simulink model "tp1_sim"  (R2018a)
settings: Solver=VariableStepAuto  StartTime=0.0  StopTime=50.0  RelTol=1e-3
values from neighbouring files (symbols this model uses):
  lambda_f = 3    [tp1.m]
  lambda_p = 5    [tp1.m]
settings Model: Creator=e1802460  LastModifiedBy=e1802460

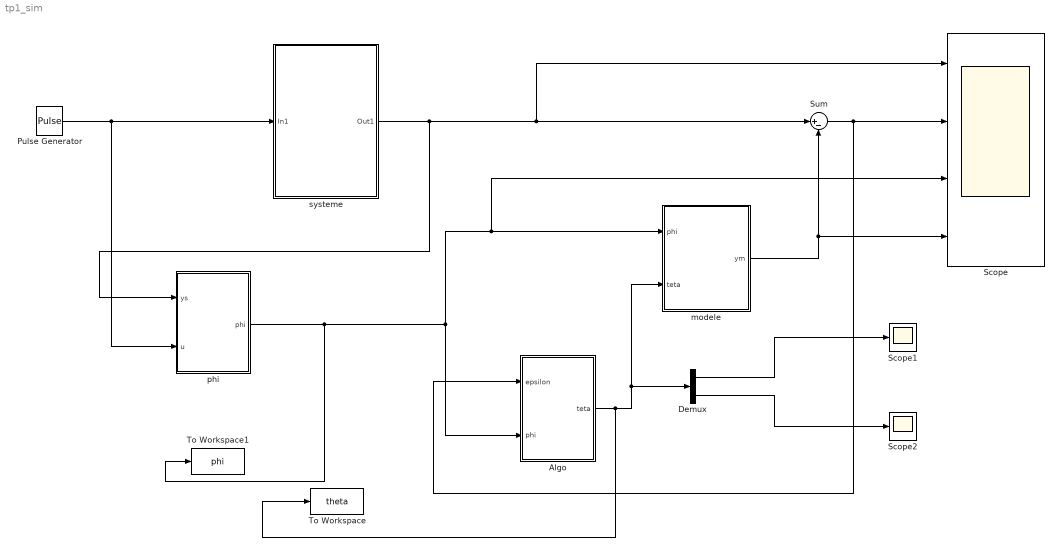
== system tp1_sim ==
  " modele " : Subsystem
  "Algo " : Subsystem
  Demux : Demux  Outputs=2
  Pulse Generator : DiscretePulseGenerator  PulseType=Time based  Period=10  PulseWidth=50
  Scope : Scope  NumInputPorts=4
  Scope1 : Scope
  Scope2 : Scope
  Sum : Sum  Inputs=|+-
  To Workspace : ToWorkspace  VariableName=theta  SaveFormat=Structure With Time  SampleTime=-1
  To Workspace1 : ToWorkspace  VariableName=phi  SaveFormat=Structure With Time  SampleTime=-1
  phi : Subsystem
  "systeme " : Subsystem
  wires:
  "systeme "/1(Out1) -> phi/1(ys), Scope/1, Sum/1
  Pulse Generator/1 -> phi/2(u), "systeme "/1(In1)
  " modele "/1(ym) -> Scope/4, Sum/2
  Sum/1 -> "Algo "/1(epsilon), Scope/2
  phi/1(phi) -> To Workspace1/1, "Algo "/2("phi "), Scope/3, " modele "/1(phi)
  "Algo "/1(teta) -> To Workspace/1, Demux/1, " modele "/2(teta)
  Demux/1 -> Scope1/1
  Demux/2 -> Scope2/1

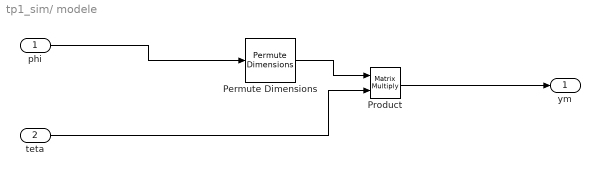
== system tp1_sim/ modele  ==
  phi : Inport
  teta : Inport  Port=2
  Permute Dimensions : PermuteDimensions
  Product : Product  Multiplication=Matrix(*)
  ym : Outport
  wires:
  Permute Dimensions/1 -> Product/1
  phi/1 -> Permute Dimensions/1
  Product/1 -> ym/1
  teta/1 -> Product/2

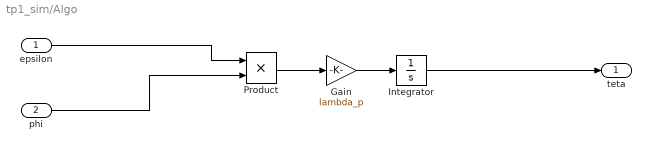
== system tp1_sim/Algo  ==
  epsilon : Inport
  "phi " : Inport  Port=2
  Gain : Gain  Gain=lambda_p
  Integrator : Integrator  InitialCondition=[0,0]
  Product : Product
  teta : Outport
  wires:
  epsilon/1 -> Product/1
  Integrator/1 -> teta/1
  "phi "/1 -> Product/2
  Product/1 -> Gain/1
  Gain/1 -> Integrator/1

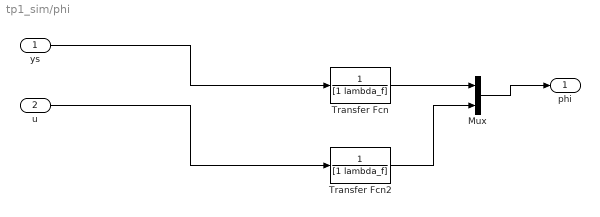
== system tp1_sim/phi ==
  ys : Inport
  u : Inport  Port=2
  Mux : Mux  Inputs=2
  Transfer Fcn : TransferFcn  Denominator=[1 lambda_f]
  Transfer Fcn2 : TransferFcn  Denominator=[1 lambda_f]
  phi : Outport
  wires:
  ys/1 -> Transfer Fcn/1
  Transfer Fcn/1 -> Mux/1
  u/1 -> Transfer Fcn2/1
  Transfer Fcn2/1 -> Mux/2
  Mux/1 -> phi/1

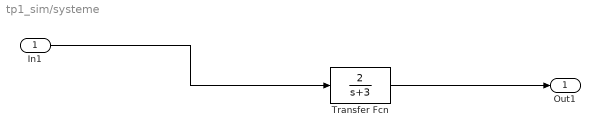
== system tp1_sim/systeme  ==
  In1 : Inport
  Transfer Fcn : TransferFcn  Numerator=[2]  Denominator=[1 3]
  Out1 : Outport
  wires:
  In1/1 -> Transfer Fcn/1
  Transfer Fcn/1 -> Out1/1
